simulink model "blockdemo"  (Simulink 6.3)
settings: Solver=ode45  StartTime=0.0  StopTime=4e-6  RelTol=1e-3
InitFcn:
  | %% DSPBuilder Start
  | alt_dspbuilder_update_model(bdroot)
  | %% DSPBuilder End
libraries: allblocks_alteradspbuilder2 x9
settings Model: Creator=cpurcell  LastModifiedBy=delphick
settings DebuggingCC: MultiTaskDSMMsg=error

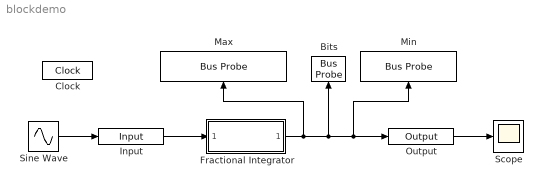
== system blockdemo ==
  Bits : allblocks_alteradspbuilder2/Bus Probe  Orientation=up  display=Maximum number of integer bits required during simulation  max_value=33.3298797607421875  min_value=-.0068359375  max_bits=7
  Clock : allblocks_alteradspbuilder2/Clock  ClockPeriod=20  ClockPeriodUnit=ns  SampleTime=20e-9  SimulationStartCycle=5  PhaseOffset=0  Reset=aclr  Export=off
  Fractional Integrator : Subsystem
  Input : allblocks_alteradspbuilder2/Input  iofile=C:\workspace_clean\Documentation\DesignExamples\Tutorials\UnitBlocks\AltLab\BusProbe\tb_blockdemo\blockdemo_Input.salt  BusType=Signed Fractional  bwl=2  bwr=16  SpecifyClock=off  PORTTYPE=Input
  Max : allblocks_alteradspbuilder2/Bus Probe  Orientation=up  display=Maximum value reached during simulation  max_value=33.3298797607421875  min_value=-.0068359375  max_bits=7
  Min : allblocks_alteradspbuilder2/Bus Probe  Orientation=up  display=Minimum value reached during simulation  max_value=33.3298797607421875  min_value=-.0068359375  max_bits=7
  Output : allblocks_alteradspbuilder2/Output  iofile=C:\workspace_clean\Documentation\DesignExamples\Tutorials\UnitBlocks\AltLab\BusProbe\tb_blockdemo\blockdemo_Output.capture  BusType=Signed Fractional  bwl=7  bwr=16  PORTTYPE=Output
  Scope : Scope
      settings: TimeRange=4e-006  YMax=40
  Sine Wave : Sin  Frequency=3e6  SampleTime=20e-9
  wires:
  Sine Wave/1 -> Input/1
  Input/1 -> Fractional Integrator/1(d[2][16])
  Fractional Integrator/1(q[14][16]) -> Bits/1, Output/1, Min/1, Max/1
  Output/1 -> Scope/1

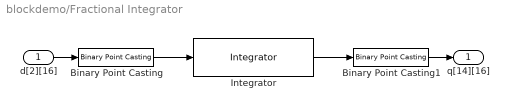
== system blockdemo/Fractional Integrator ==
  d[2][16] : Inport
  Binary Point Casting : allblocks_alteradspbuilder2/Binary Point Casting  BusType=Signed Fractional  bwl=2  bwr=16  OutputPointPosition=0
  Binary Point Casting1 : allblocks_alteradspbuilder2/Binary Point Casting  BusType=Signed Fractional  bwl=30  bwr=0  OutputPointPosition=16
  Integrator : allblocks_alteradspbuilder2/Integrator  bwl=30  depth=1  use_ena=off  use_sclr=off
  q[14][16] : Outport
  wires:
  Binary Point Casting/1 -> Integrator/1
  Integrator/1 -> Binary Point Casting1/1
  d[2][16]/1 -> Binary Point Casting/1
  Binary Point Casting1/1 -> q[14][16]/1
